simulink model "suspensionIDTest"  (R2015a)
settings: Solver=ode23t  StartTime=0.0  StopTime=10  RelTol=1e-3
PreLoadFcn:
  | load carParams;
  | 
  | % Create blank state-space placeholder.
  | changeMe = ss(0,0,0,0);
values from neighbouring files (symbols this model uses):
  b1 = 2500    [carParams.mat]
  b2 = 15000    [carParams.mat]
libraries: fl_lib x9, nesl_utility x3, cstblocks x1
settings Model: Creator=scastro  LastModifiedBy=chahn
settings DataIOCC: LimitDataPoints=off  OutputTimes=0:0.001:60
settings SimscapeCC: SimscapeLogType=all  SimscapeLogDataHistory=10000

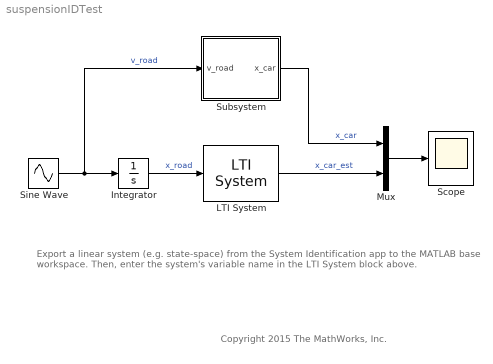
== system suspensionIDTest ==
  note: Export a linear system (e.g. state-space) from the System Identification app to the MATLAB base workspace.
      |
      | Then, enter the system's variable name in the LTI System block above.
  note: Copyright 2015 The MathWorks, Inc.
  Integrator : Integrator
  LTI System : cstblocks/LTI System  sys=changeMe  IC=[]
  Mux : Mux  Inputs=2
  Scope : Scope
      settings: ShowLegends=on  TimeRange=10  YMin=-0.15  YMax=0.15
  Sine Wave : Sin  Amplitude=250  Frequency=100  Phase=pi/2  SampleTime=0
  Subsystem : Subsystem
  wires:
  Integrator/1 -> LTI System/1  "x_road"
  LTI System/1 -> Mux/2  "x_car_est"
  Subsystem/1(x_car) -> Mux/1  "x_car"
  Mux/1 -> Scope/1
  Sine Wave/1 -> Subsystem/1(v_road), Integrator/1  "v_road"

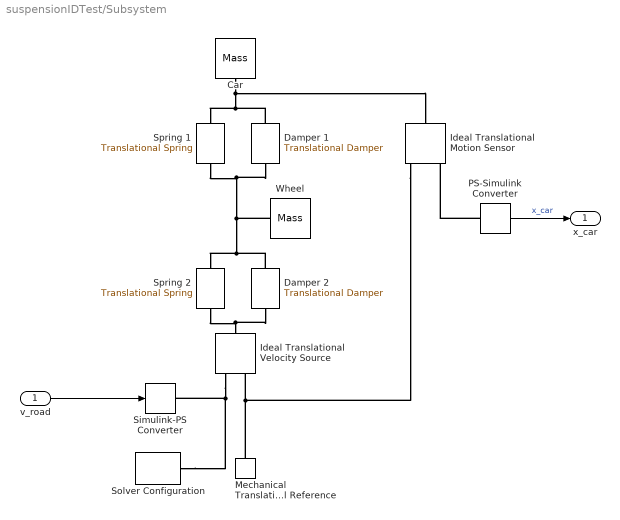
== system suspensionIDTest/Subsystem ==
  v_road : Inport
  Car : fl_lib/Mechanical/Translational Elements/Mass  mass=mCar kg  v_specify=on  v_priority=High  v=0 m/s  f_specify=off  f_priority=High  f=0 N
  Damper 1 : fl_lib/Mechanical/Translational Elements/Translational Damper  D=b1 N/(m/s)  v_specify=off  v_priority=High  v=0 m/s  f_specify=off  f_priority=High  f=0 N
  Damper 2 : fl_lib/Mechanical/Translational Elements/Translational Damper  D=b2 N/(m/s)  v_specify=off  v_priority=High  v=0 m/s  f_specify=off  f_priority=High  f=0 N
  Ideal Translational Motion Sensor : fl_lib/Mechanical/Mechanical Sensors/Ideal Translational Motion Sensor  offset=0 m
  Ideal Translational Velocity Source : fl_lib/Mechanical/Mechanical Sources/Ideal Translational Velocity Source
  Mechanical Translational Reference : fl_lib/Mechanical/Translational Elements/Mechanical Translational Reference
  PS-Simulink Converter : nesl_utility/PS-Simulink Converter  PhysicalDomain=network_engine_domain  SubClassName=ps_output  LeftPortType=input  RightPortType=output  PseudoPeriodic=off  Frequencies=[]  Unit=cm  AffineConversion=off
  Simulink-PS Converter : nesl_utility/Simulink-PS Converter  PhysicalDomain=network_engine_domain  SubClassName=ps_input  LeftPortType=input  RightPortType=output  PseudoPeriodic=off  Frequencies=[]  NoiseDistribution=none  NoiseParameters=[]  Unit=cm/s  AffineConversion=off  InputFiltering=off  SimscapeFilterOrder=1  InputFilterTimeConstant=0.001  UdotUserProvided=1
  Solver Configuration : nesl_utility/Solver Configuration  PhysicalDomain=network_engine_domain  SubClassName=solver  LeftPortType=input  RightPortType=generic  Accelerate=off  Tones=[]  Harmonics=[]  SimulateNoise=off  Profile=off  UseLocalSampling=off  EnableSwitchedLinearOptims=on  FrequencyDomain=off  UseCCode=off  RelTol=0.001  AbsTol=1e-06  MinStep=1e-09  ToWorkspace=off  RevertToSquareIcSolve=off  NumHomotopyIterations=100  DoDC=off  ResidualTolerance=1e-09  UseLocalSolver=off  LocalSolverChoice=NE_BACKWARD_EULER_ADVANCER  LocalSolverSampleTime=0.001  DoFixedCost=off  MaxNonlinIter=3  MaxModeIter=2  LinearAlgebra=Sparse  DelaysMemoryBudget=1024  AutomaticFiltering=on  FilteringTimeConstant=0.001
  Spring 1 : fl_lib/Mechanical/Translational Elements/Translational Spring  spr_rate=k1 N/m  v_specify=off  v_priority=High  v=0 m/s  f_specify=off  f_priority=High  f=0 N  x_specify=off  x_priority=High  x=0 m
  Spring 2 : fl_lib/Mechanical/Translational Elements/Translational Spring  spr_rate=k2 N/m  v_specify=off  v_priority=High  v=0 m/s  f_specify=off  f_priority=High  f=0 N  x_specify=off  x_priority=High  x=0 m
  Wheel : fl_lib/Mechanical/Translational Elements/Mass  mass=mWheel kg  v_specify=off  v_priority=High  v=0 m/s  f_specify=off  f_priority=High  f=0 N
  x_car : Outport
  wires:
  PS-Simulink Converter/1 -> x_car/1  "x_car"
  v_road/1 -> Simulink-PS Converter/1
  connections:
  Ideal Translational Velocity Source/RConn1 -- Solver Configuration/RConn1 -- Simulink-PS Converter/RConn1
  Mechanical Translational Reference/LConn1 -- Ideal Translational Motion Sensor/RConn1 -- Ideal Translational Velocity Source/RConn2
  PS-Simulink Converter/LConn1 -- Ideal Translational Motion Sensor/RConn3
  Damper 1/RConn1 -- Spring 1/RConn1 -- Damper 2/LConn1 -- Spring 2/LConn1 -- Wheel/LConn1
  Spring 2/RConn1 -- Damper 2/RConn1 -- Ideal Translational Velocity Source/LConn1
  Spring 1/LConn1 -- Ideal Translational Motion Sensor/LConn1 -- Car/LConn1 -- Damper 1/LConn1
